simulink model "testEMplanner_cs"  (R2020b)
settings: Solver=FixedStepAuto  StartTime=0.0  StopTime=inf  FixedStep=1/1000  RelTol=1e-3
PreLoadFcn:
  | mbxruntime.callbacks.PreLoadFcn(bdroot);
PostLoadFcn:
  | mbxruntime.callbacks.PostLoadFcn(bdroot);
InitFcn:
  | mbxruntime.callbacks.InitFcn(bdroot);
StartFcn:
  | mbxruntime.callbacks.StartFcn(bdroot);
StopFcn:
  | mbxruntime.callbacks.StopFcn(bdroot);
model workspace: external: MAT-File testEMplanner_cs_hws.mat (data not in the file)
undefined symbols (not defined in the file): aubr, c_factor, cf, cr, DiscIntNeverNeededParam, global_path_x, global_path_y, KD_PID_distance, KD_PID_speed, KI_PID_distance, KI_PID_speed, KP_PID_distance, KP_PID_speed, la, lb, LQR_K1, LQR_K2, LQR_K3, LQR_K4, m, rack_displacement, right_wheel_ground, tablebr, vubr, vx_break_point
libraries: PreScanSimulinkLibrary x38, Solver_SF x1
(part 1 of 16)
CloseFcn:
  | mbxruntime.callbacks.CloseFcn(bdroot);
settings Model: Creator=PRESCAN  LastModifiedBy=iJeju
settings DataIOCC: LimitDataPoints=on  SaveFormat=Array  SignalLoggingSaveFormat=ModelDataLogs  ReturnWorkspaceOutputs=off
settings OptimizationCC: ExpressionDepthLimit=2147483647  ZeroExternalMemoryAtStartup=off  ZeroInternalMemoryAtStartup=off  InitFltsAndDblsToZero=on  LifeSpan=inf
settings DebuggingCC: SaveWithParameterizedLinksMsg=none  UnderspecifiedInitializationDetection=Classic  MergeDetectMultiDrivingBlocksExec=none  SignalResolutionControl=TryResolveAllWithWarning  MultiTaskDSMMsg=warning  MultiTaskCondExecSysMsg=none  UnderSpecifiedDataTypeMsg=warning  FcnCallInpInsideContextMsg=warning  StateNameClashWarn=warning  SFUnexpectedBacktrackingDiag=warning  SFNoUnconditionalDefaultTransitionDiag=warning  SFExecutionAtInitializationDiag=none  UnderSpecifiedDimensionMsg=warning  ArithmeticOperatorsInVariantConditions=warning
settings HardwareCC: ProdBitPerPointer=32  ProdBitPerSizeT=32  ProdBitPerPtrDiffT=32  ProdLargestAtomicFloat=None  ProdIntDivRoundTo=Undefined  ProdEndianess=Unspecified  ProdWordSize=32  ProdHWDeviceType=32-bit Generic
settings ModelReferenceCC: UpdateModelReferenceTargets=IfOutOfDate  PropagateSignalLabelsOutOfModel=off
settings SFSimCC: SimUseLocalCustomCode=off  SimParseCustomCode=off  CustomCodeUndefinedFunction=UseInterfaceOnly
settings SFSimCC: SimCustomHeaderCode=|
  | #include "prescan.h"
  | #include "prescan_platform.h"
settings RTWCC: RTWUseLocalCustomCode=off  TargetLang=C++
settings CodeAppCC: StateflowObjectComments=on
settings GRTTargetCC: TargetFcnLib=ansi_tfl_tmw.mat  TargetLangStandard=C++03 (ISO)  CodeInterfacePackaging=C++ class
settings ConfigComp: CovMetricSettings=dw  CovSaveCumulativeToWorkspaceVar=on  CovSaveSingleToWorkspaceVar=on  CovExternalEMLEnable=off

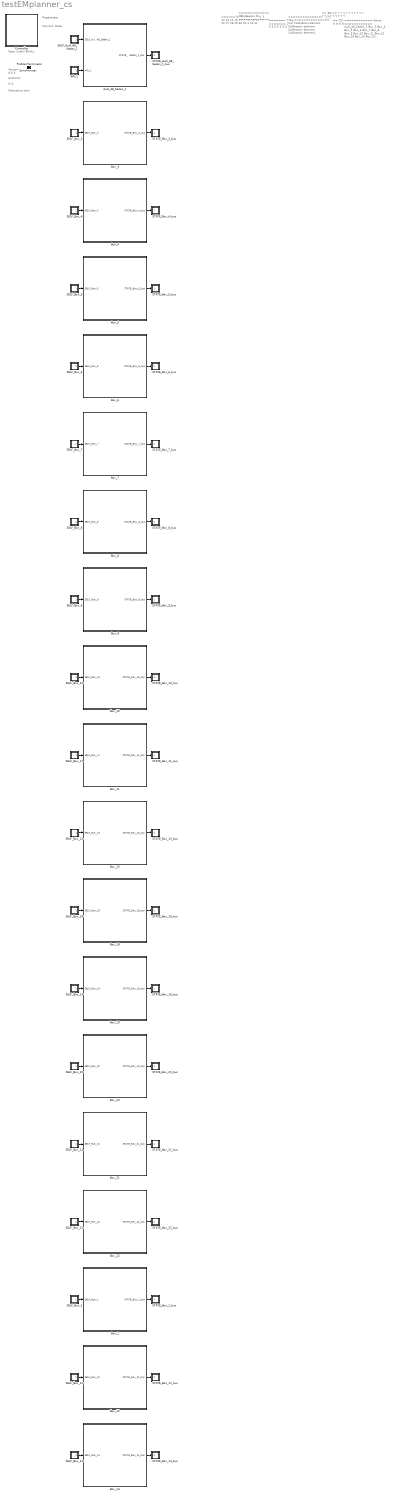
== system testEMplanner_cs ==
  note: Regenerate
  note: Simulink Mode
  note: Open Useful Blocks
  note: 8.6.0
  note: Version:
  note: Author(s):
  note: N.A.
  note: Descriptive text:
  note: ======
      | Num ID
      | ======
      | 3
      | 12
      | 13
      | 14
      | 15
      | 16
      | 17
      | 18
      | 19
      | 20
      | 22
      | 27
      | 28
      | 29
      | 30
      | 31
      | 4
      | 10
      | 21
  note: =============
      | OBU-Beacon ID
      | =============
  note: =======
      | Type ID
      | =======
      | 1
      | 5
      | 5
      | 5
      | 5
      | 5
      | 5
      | 5
      | 5
      | 5
      | 5
      | 5
      | 5
      | 5
      | 5
      | 5
      | 5
      | 5
      | 5
  note: ===============
      | Type Tag
      | ===============
      | Car
      | Calibration element
      | Calibration element
      | Calibration element
      | Calibration element
      | Calibration element
      | Calibration element
      | Calibration element
      | Calibration element
      | Calibration element
      | Calibration element
      | Calibration element
      | Calibration element
      | Calibration element
      | Calibration element
      | Calibration element
      | Calibration element
      | Calibration element
      | Calibration element
  note: ==
      | SD
      | ==
      | Y
      | Y
      | Y
      | Y
      | Y
      | Y
      | Y
      | Y
      | Y
      | Y
      | Y
      | Y
      | Y
      | Y
      | Y
      | Y
      | Y
      | Y
      | Y
  note: ==
      | CD
      | ==
      | N
      | N
      | N
      | N
      | N
      | N
      | N
      | N
      | N
      | N
      | N
      | N
      | N
      | N
      | N
      | N
      | N
      | N
      | N
  note: ============
      | Name
      | ============
      | Audi_A8_Sedan_1
      | Box_3
      | Box_4
      | Box_5
      | Box_6
      | Box_7
      | Box_8
      | Box_9
      | Box_10
      | Box_11
      | Box_13
      | Box_18
      | Box_19
      | Box_20
      | Box_21
      | Box_22
      | Box_1
      | Box_12
      | Box_14
  AIR_1 : Subsystem  Tag=sensor/AIR  Priority=3  LoadFcn=load('PrescanAIRSensorData.mat');load('PrescanAIRSensorMessage.mat')  mask(PreScan Source Block: Actor Independent Receiver (AIR)){}
      mask help:
      | The Actor Information Receiver sensor provides a fast, simple and generic detection solution which is not tied up to a specific technology. The AIR detects the intersection point of the bounding box with the straight line from the sensor axis system to the middle of the bounding box.
      |
      | For more information, please click Help.
      settings: OpenFcn=open_system([gcb '/Sensor'],'mask')
      mask Help: eval('openHelp(413)')
      mask Display: image(imread('AIR.png'))
  Audi_A8_Sedan_1 : Subsystem  Tag=WorldObjectSubSystem  InitFcn=UniqueId = '15';
      mask init:
      | modelPath = GenericModelHelper.getGenericModelFilePath('ModelDepo','Vehicles\Audi_A8\Audi_A8.pgmb','d771622804618130053427da08a6d484');imagePath = GenericModelHelper.getCompilationPicture(modelPath, 'Audi_A8_HighPoly.png');
      mask Display: image(imread(imagePath));color('white');text(0, 0, ' ID=3\n')
  Box_1 : Subsystem  Tag=WorldObjectSubSystem  InitFcn=|
      | UniqueId = '143';
      | UniqueId = '276';
      mask init:
      | imagePath=which('Box.jpg');
      mask Display: image(imread(imagePath));color('white');text(0, 0, ' ID=4\n')
  Box_10 : Subsystem  Tag=WorldObjectSubSystem  InitFcn=UniqueId = '177';
      mask init:
      | imagePath=which('Box.jpg');
      mask Display: image(imread(imagePath));color('white');text(0, 0, ' ID=19\n')
  Box_11 : Subsystem  Tag=WorldObjectSubSystem  InitFcn=UniqueId = '178';
      mask init:
      | imagePath=which('Box.jpg');
      mask Display: image(imread(imagePath));color('white');text(0, 0, ' ID=20\n')
  Box_12 : Subsystem  Tag=WorldObjectSubSystem  InitFcn=|
      | UniqueId = '179';
      | UniqueId = '277';
      mask init:
      | imagePath=which('Box.jpg');
      mask Display: image(imread(imagePath));color('white');text(0, 0, ' ID=10\n')
  Box_13 : Subsystem  Tag=WorldObjectSubSystem  InitFcn=UniqueId = '182';
      mask init:
      | imagePath=which('Box.jpg');
      mask Display: image(imread(imagePath));color('white');text(0, 0, ' ID=22\n')
  Box_14 : Subsystem  Tag=WorldObjectSubSystem  InitFcn=|
      | UniqueId = '183';
      | UniqueId = '281';
      mask init:
      | imagePath=which('Box.jpg');
      mask Display: image(imread(imagePath));color('white');text(0, 0, ' ID=21\n')
  Box_18 : Subsystem  Tag=WorldObjectSubSystem  InitFcn=UniqueId = '195';
      mask init:
      | imagePath=which('Box.jpg');
      mask Display: image(imread(imagePath));color('white');text(0, 0, ' ID=27\n')
  Box_19 : Subsystem  Tag=WorldObjectSubSystem  InitFcn=UniqueId = '196';
      mask init:
      | imagePath=which('Box.jpg');
      mask Display: image(imread(imagePath));color('white');text(0, 0, ' ID=28\n')
  Box_20 : Subsystem  Tag=WorldObjectSubSystem  InitFcn=UniqueId = '197';
      mask init:
      | imagePath=which('Box.jpg');
      mask Display: image(imread(imagePath));color('white');text(0, 0, ' ID=29\n')
  Box_21 : Subsystem  Tag=WorldObjectSubSystem  InitFcn=UniqueId = '198';
      mask init:
      | imagePath=which('Box.jpg');
      mask Display: image(imread(imagePath));color('white');text(0, 0, ' ID=30\n')
  Box_22 : Subsystem  Tag=WorldObjectSubSystem  InitFcn=UniqueId = '199';
      mask init:
      | imagePath=which('Box.jpg');
      mask Display: image(imread(imagePath));color('white');text(0, 0, ' ID=31\n')
  Box_3 : Subsystem  Tag=WorldObjectSubSystem  InitFcn=UniqueId = '170';
      mask init:
      | imagePath=which('Box.jpg');
      mask Display: image(imread(imagePath));color('white');text(0, 0, ' ID=12\n')
  Box_4 : Subsystem  Tag=WorldObjectSubSystem  InitFcn=UniqueId = '171';
      mask init:
      | imagePath=which('Box.jpg');
      mask Display: image(imread(imagePath));color('white');text(0, 0, ' ID=13\n')
  Box_5 : Subsystem  Tag=WorldObjectSubSystem  InitFcn=UniqueId = '172';
      mask init:
      | imagePath=which('Box.jpg');
      mask Display: image(imread(imagePath));color('white');text(0, 0, ' ID=14\n')
  Box_6 : Subsystem  Tag=WorldObjectSubSystem  InitFcn=UniqueId = '173';
      mask init:
      | imagePath=which('Box.jpg');
      mask Display: image(imread(imagePath));color('white');text(0, 0, ' ID=15\n')
  Box_7 : Subsystem  Tag=WorldObjectSubSystem  InitFcn=UniqueId = '174';
      mask init:
      | imagePath=which('Box.jpg');
      mask Display: image(imread(imagePath));color('white');text(0, 0, ' ID=16\n')
  Box_8 : Subsystem  Tag=WorldObjectSubSystem  InitFcn=UniqueId = '175';
      mask init:
      | imagePath=which('Box.jpg');
      mask Display: image(imread(imagePath));color('white');text(0, 0, ' ID=17\n')
  Box_9 : Subsystem  Tag=WorldObjectSubSystem  InitFcn=UniqueId = '176';
      mask init:
      | imagePath=which('Box.jpg');
      mask Display: image(imread(imagePath));color('white');text(0, 0, ' ID=18\n')
  Controller : Subsystem  Description=73E1798A8DDC6C7523B87793F8265ADBA4092B5E929CBACDAD4A169A3E9AE576  Priority=-1  LoadFcn=load PreScanControllerData  mask(PreScan Simulation Controller){prescanversion='8.6.0', ModelReferencing=off, TimeStep=50/1000, ControlMode=0, PreScanExecutionMode=on, ControllerCount=0, ControllerIndex=0, ControllerOptions=''}
      mask prompts: prescanversion "PreScan Version"; ModelReferencing "Use Model Referencing"; TimeStep "Upload Period [s]"; ControlMode "Control Mode"; PreScanExecutionMode "Execution Mode"; ControllerCount "Controller Count"; ControllerIndex "Controller Index"; ControllerOptions "Controller Options"
      mask help:
      | Please do not remove this block from the compilation sheet,
      | as it connects the model to the PreScan environment.
      mask init:
      | model = bdroot(gcb);
      | ExperimentFile = mbxruntime.findExperimentFile(model,true); %relative path
      | 
      | [d1, d2, d3, prescandata] = prescan_Settings();
      | ModelDepo = fullfile(prescandata,'ModelDepo'); 
      | 
      | RTmode = mbxruntime.getRTMode(model);
      | 
      | SimulationMode = get_param(bdroot,'SimulationMode');
      | if strcmp(SimulationMode, 'rapid-accelerator')
      |     SimulationMode = 'external';
      | end
      | TargetName = get_param(bdroot,'SystemTargetFile');
      settings: ModelCloseFcn=assignin('base',['model_closed_' bdroot],true);
      mask Help: eval('openHelp(812)')
      mask Display: image(imread('prescanlogo.ico'))
  PreScanTerminator : Subsystem  Tag=PreScanTerminator  Priority=999  LoadFcn=load PrescanTerminatorData  mask(PreScan Simulation Terminator){TimeStep=50/1000}
      mask prompts: TimeStep "Upload Period [s]"
      mask help:
      | Please do not remove this block from the compilation sheet as it
      | connects the model to the PreScan environment.
      mask Help: eval('openHelp(812)')
      mask Display: image(imread('prescanlogo.ico'))
  SELF_Audi_A8_Sedan_1 : Subsystem  Tag=sensor/SelfPort  Priority=3  LoadFcn=load('PreScanSelfSensorData.mat')  mask(PreScan Source Block: SELF){}
      mask help:
      | The SELF port shows (state) information of the actor itself. The outputs are position in the experiment's axis system and the GPS coordinates, and the object's absolute velocity and compass heading.
      |
      | For more information, please click Help.
      settings: OpenFcn=open_system([gcb '/Sensor'],'mask')
      mask Help: eval('openHelp(462)')
      mask Display: image(imread('GPS.png'))
  SELF_Box_1 : Subsystem  Tag=sensor/SelfPort  Priority=3  LoadFcn=load('PreScanSelfSensorData.mat')  mask(PreScan Source Block: SELF){}
      mask help:
      | The SELF port shows (state) information of the actor itself. The outputs are position in the experiment's axis system and the GPS coordinates, and the object's absolute velocity and compass heading.
      |
      | For more information, please click Help.
      settings: OpenFcn=open_system([gcb '/Sensor'],'mask')
      mask Help: eval('openHelp(462)')
      mask Display: image(imread('GPS.png'))
  SELF_Box_10 : Subsystem  Tag=sensor/SelfPort  Priority=3  LoadFcn=load('PreScanSelfSensorData.mat')  mask(PreScan Source Block: SELF){}
      mask help:
      | The SELF port shows (state) information of the actor itself. The outputs are position in the experiment's axis system and the GPS coordinates, and the object's absolute velocity and compass heading.
      |
      | For more information, please click Help.
      settings: OpenFcn=open_system([gcb '/Sensor'],'mask')
      mask Help: eval('openHelp(462)')
      mask Display: image(imread('GPS.png'))
  SELF_Box_11 : Subsystem  Tag=sensor/SelfPort  Priority=3  LoadFcn=load('PreScanSelfSensorData.mat')  mask(PreScan Source Block: SELF){}
      mask help:
      | The SELF port shows (state) information of the actor itself. The outputs are position in the experiment's axis system and the GPS coordinates, and the object's absolute velocity and compass heading.
      |
      | For more information, please click Help.
      settings: OpenFcn=open_system([gcb '/Sensor'],'mask')
      mask Help: eval('openHelp(462)')
      mask Display: image(imread('GPS.png'))
  SELF_Box_12 : Subsystem  Tag=sensor/SelfPort  Priority=3  LoadFcn=load('PreScanSelfSensorData.mat')  mask(PreScan Source Block: SELF){}
      mask help:
      | The SELF port shows (state) information of the actor itself. The outputs are position in the experiment's axis system and the GPS coordinates, and the object's absolute velocity and compass heading.
      |
      | For more information, please click Help.
      settings: OpenFcn=open_system([gcb '/Sensor'],'mask')
      mask Help: eval('openHelp(462)')
      mask Display: image(imread('GPS.png'))
  SELF_Box_13 : Subsystem  Tag=sensor/SelfPort  Priority=3  LoadFcn=load('PreScanSelfSensorData.mat')  mask(PreScan Source Block: SELF){}
      mask help:
      | The SELF port shows (state) information of the actor itself. The outputs are position in the experiment's axis system and the GPS coordinates, and the object's absolute velocity and compass heading.
      |
      | For more information, please click Help.
      settings: OpenFcn=open_system([gcb '/Sensor'],'mask')
      mask Help: eval('openHelp(462)')
      mask Display: image(imread('GPS.png'))
  SELF_Box_14 : Subsystem  Tag=sensor/SelfPort  Priority=3  LoadFcn=load('PreScanSelfSensorData.mat')  mask(PreScan Source Block: SELF){}
      mask help:
      | The SELF port shows (state) information of the actor itself. The outputs are position in the experiment's axis system and the GPS coordinates, and the object's absolute velocity and compass heading.
      |
      | For more information, please click Help.
      settings: OpenFcn=open_system([gcb '/Sensor'],'mask')
      mask Help: eval('openHelp(462)')
      mask Display: image(imread('GPS.png'))
  SELF_Box_18 : Subsystem  Tag=sensor/SelfPort  Priority=3  LoadFcn=load('PreScanSelfSensorData.mat')  mask(PreScan Source Block: SELF){}
      mask help:
      | The SELF port shows (state) information of the actor itself. The outputs are position in the experiment's axis system and the GPS coordinates, and the object's absolute velocity and compass heading.
      |
      | For more information, please click Help.
      settings: OpenFcn=open_system([gcb '/Sensor'],'mask')
      mask Help: eval('openHelp(462)')
      mask Display: image(imread('GPS.png'))
  SELF_Box_19 : Subsystem  Tag=sensor/SelfPort  Priority=3  LoadFcn=load('PreScanSelfSensorData.mat')  mask(PreScan Source Block: SELF){}
      mask help:
      | The SELF port shows (state) information of the actor itself. The outputs are position in the experiment's axis system and the GPS coordinates, and the object's absolute velocity and compass heading.
      |
      | For more information, please click Help.
      settings: OpenFcn=open_system([gcb '/Sensor'],'mask')
      mask Help: eval('openHelp(462)')
      mask Display: image(imread('GPS.png'))
  SELF_Box_20 : Subsystem  Tag=sensor/SelfPort  Priority=3  LoadFcn=load('PreScanSelfSensorData.mat')  mask(PreScan Source Block: SELF){}
      mask help:
      | The SELF port shows (state) information of the actor itself. The outputs are position in the experiment's axis system and the GPS coordinates, and the object's absolute velocity and compass heading.
      |
      | For more information, please click Help.
      settings: OpenFcn=open_system([gcb '/Sensor'],'mask')
      mask Help: eval('openHelp(462)')
      mask Display: image(imread('GPS.png'))
  SELF_Box_21 : Subsystem  Tag=sensor/SelfPort  Priority=3  LoadFcn=load('PreScanSelfSensorData.mat')  mask(PreScan Source Block: SELF){}
      mask help:
      | The SELF port shows (state) information of the actor itself. The outputs are position in the experiment's axis system and the GPS coordinates, and the object's absolute velocity and compass heading.
      |
      | For more information, please click Help.
      settings: OpenFcn=open_system([gcb '/Sensor'],'mask')
      mask Help: eval('openHelp(462)')
      mask Display: image(imread('GPS.png'))
  SELF_Box_22 : Subsystem  Tag=sensor/SelfPort  Priority=3  LoadFcn=load('PreScanSelfSensorData.mat')  mask(PreScan Source Block: SELF){}
      mask help:
      | The SELF port shows (state) information of the actor itself. The outputs are position in the experiment's axis system and the GPS coordinates, and the object's absolute velocity and compass heading.
      |
      | For more information, please click Help.
      settings: OpenFcn=open_system([gcb '/Sensor'],'mask')
      mask Help: eval('openHelp(462)')
      mask Display: image(imread('GPS.png'))
  SELF_Box_3 : Subsystem  Tag=sensor/SelfPort  Priority=3  LoadFcn=load('PreScanSelfSensorData.mat')  mask(PreScan Source Block: SELF){}
      mask help:
      | The SELF port shows (state) information of the actor itself. The outputs are position in the experiment's axis system and the GPS coordinates, and the object's absolute velocity and compass heading.
      |
      | For more information, please click Help.
      settings: OpenFcn=open_system([gcb '/Sensor'],'mask')
      mask Help: eval('openHelp(462)')
      mask Display: image(imread('GPS.png'))
  SELF_Box_4 : Subsystem  Tag=sensor/SelfPort  Priority=3  LoadFcn=load('PreScanSelfSensorData.mat')  mask(PreScan Source Block: SELF){}
      mask help:
      | The SELF port shows (state) information of the actor itself. The outputs are position in the experiment's axis system and the GPS coordinates, and the object's absolute velocity and compass heading.
      |
      | For more information, please click Help.
      settings: OpenFcn=open_system([gcb '/Sensor'],'mask')
      mask Help: eval('openHelp(462)')
      mask Display: image(imread('GPS.png'))
  SELF_Box_5 : Subsystem  Tag=sensor/SelfPort  Priority=3  LoadFcn=load('PreScanSelfSensorData.mat')  mask(PreScan Source Block: SELF){}
      mask help:
      | The SELF port shows (state) information of the actor itself. The outputs are position in the experiment's axis system and the GPS coordinates, and the object's absolute velocity and compass heading.
      |
      | For more information, please click Help.
      settings: OpenFcn=open_system([gcb '/Sensor'],'mask')
      mask Help: eval('openHelp(462)')
      mask Display: image(imread('GPS.png'))
  SELF_Box_6 : Subsystem  Tag=sensor/SelfPort  Priority=3  LoadFcn=load('PreScanSelfSensorData.mat')  mask(PreScan Source Block: SELF){}
      mask help:
      | The SELF port shows (state) information of the actor itself. The outputs are position in the experiment's axis system and the GPS coordinates, and the object's absolute velocity and compass heading.
      |
      | For more information, please click Help.
      settings: OpenFcn=open_system([gcb '/Sensor'],'mask')
      mask Help: eval('openHelp(462)')
      mask Display: image(imread('GPS.png'))
  SELF_Box_7 : Subsystem  Tag=sensor/SelfPort  Priority=3  LoadFcn=load('PreScanSelfSensorData.mat')  mask(PreScan Source Block: SELF){}
      mask help:
      | The SELF port shows (state) information of the actor itself. The outputs are position in the experiment's axis system and the GPS coordinates, and the object's absolute velocity and compass heading.
      |
      | For more information, please click Help.
      settings: OpenFcn=open_system([gcb '/Sensor'],'mask')
      mask Help: eval('openHelp(462)')
      mask Display: image(imread('GPS.png'))
  SELF_Box_8 : Subsystem  Tag=sensor/SelfPort  Priority=3  LoadFcn=load('PreScanSelfSensorData.mat')  mask(PreScan Source Block: SELF){}
      mask help:
      | The SELF port shows (state) information of the actor itself. The outputs are position in the experiment's axis system and the GPS coordinates, and the object's absolute velocity and compass heading.
      |
      | For more information, please click Help.
      settings: OpenFcn=open_system([gcb '/Sensor'],'mask')
      mask Help: eval('openHelp(462)')
      mask Display: image(imread('GPS.png'))
  SELF_Box_9 : Subsystem  Tag=sensor/SelfPort  Priority=3  LoadFcn=load('PreScanSelfSensorData.mat')  mask(PreScan Source Block: SELF){}
      mask help:
      | The SELF port shows (state) information of the actor itself. The outputs are position in the experiment's axis system and the GPS coordinates, and the object's absolute velocity and compass heading.
      |
      | For more information, please click Help.
      settings: OpenFcn=open_system([gcb '/Sensor'],'mask')
      mask Help: eval('openHelp(462)')
      mask Display: image(imread('GPS.png'))
  STATE_Audi_A8_Sedan_1_bus : Subsystem  Tag=actuator/StatePort  Priority=0  LoadFcn=load('PreScanStateActuatorData.mat')  mask(PreScan Sink Block: State){}
      mask help:
      | The Actor State contains a vector signal of size (9x1), containing the following signals:
      |
      | -  Position    	(x,y,z)             	[m]
      | -  Velocity    	(vx,vy,vz)         	[m/s]
      | -  Angles       	(Roll, Pitch, Yaw)	[rad]
      |
      | The Actor state is defined in the global axis system.
      | The state is superponed on the Initial position defined in the GUI.
      |
      | For more information, please click Help.
      settings: OpenFcn=open_system([gcb '/Actuator'],'mask')
      mask Help: eval('openHelp(222)')
      mask Display: image(imread('State.png'))
  STATE_Box_10_bus : Subsystem  Tag=actuator/StatePort  Priority=0  LoadFcn=load('PreScanStateActuatorData.mat')  mask(PreScan Sink Block: State){}
      mask help:
      | The Actor State contains a vector signal of size (9x1), containing the following signals:
      |
      | -  Position    	(x,y,z)             	[m]
      | -  Velocity    	(vx,vy,vz)         	[m/s]
      | -  Angles       	(Roll, Pitch, Yaw)	[rad]
      |
      | The Actor state is defined in the global axis system.
      | The state is superponed on the Initial position defined in the GUI.
      |
      | For more information, please click Help.
      settings: OpenFcn=open_system([gcb '/Actuator'],'mask')
      mask Help: eval('openHelp(222)')
      mask Display: image(imread('State.png'))
  STATE_Box_11_bus : Subsystem  Tag=actuator/StatePort  Priority=0  LoadFcn=load('PreScanStateActuatorData.mat')  mask(PreScan Sink Block: State){}
      mask help:
      | The Actor State contains a vector signal of size (9x1), containing the following signals:
      |
      | -  Position    	(x,y,z)             	[m]
      | -  Velocity    	(vx,vy,vz)         	[m/s]
      | -  Angles       	(Roll, Pitch, Yaw)	[rad]
      |
      | The Actor state is defined in the global axis system.
      | The state is superponed on the Initial position defined in the GUI.
      |
      | For more information, please click Help.
      settings: OpenFcn=open_system([gcb '/Actuator'],'mask')
      mask Help: eval('openHelp(222)')
      mask Display: image(imread('State.png'))
  STATE_Box_12_bus : Subsystem  Tag=actuator/StatePort  Priority=0  LoadFcn=load('PreScanStateActuatorData.mat')  mask(PreScan Sink Block: State){}
      mask help:
      | The Actor State contains a vector signal of size (9x1), containing the following signals:
      |
      | -  Position    	(x,y,z)             	[m]
      | -  Velocity    	(vx,vy,vz)         	[m/s]
      | -  Angles       	(Roll, Pitch, Yaw)	[rad]
      |
      | The Actor state is defined in the global axis system.
      | The state is superponed on the Initial position defined in the GUI.
      |
      | For more information, please click Help.
      settings: OpenFcn=open_system([gcb '/Actuator'],'mask')
      mask Help: eval('openHelp(222)')
      mask Display: image(imread('State.png'))
  STATE_Box_13_bus : Subsystem  Tag=actuator/StatePort  Priority=0  LoadFcn=load('PreScanStateActuatorData.mat')  mask(PreScan Sink Block: State){}
      mask help:
      | The Actor State contains a vector signal of size (9x1), containing the following signals:
      |
      | -  Position    	(x,y,z)             	[m]
      | -  Velocity    	(vx,vy,vz)         	[m/s]
      | -  Angles       	(Roll, Pitch, Yaw)	[rad]
      |
      | The Actor state is defined in the global axis system.
      | The state is superponed on the Initial position defined in the GUI.
      |
      | For more information, please click Help.
      settings: OpenFcn=open_system([gcb '/Actuator'],'mask')
      mask Help: eval('openHelp(222)')
      mask Display: image(imread('State.png'))
  STATE_Box_14_bus : Subsystem  Tag=actuator/StatePort  Priority=0  LoadFcn=load('PreScanStateActuatorData.mat')  mask(PreScan Sink Block: State){}
      mask help:
      | The Actor State contains a vector signal of size (9x1), containing the following signals:
      |
      | -  Position    	(x,y,z)             	[m]
      | -  Velocity    	(vx,vy,vz)         	[m/s]
      | -  Angles       	(Roll, Pitch, Yaw)	[rad]
      |
      | The Actor state is defined in the global axis system.
      | The state is superponed on the Initial position defined in the GUI.
      |
      | For more information, please click Help.
      settings: OpenFcn=open_system([gcb '/Actuator'],'mask')
      mask Help: eval('openHelp(222)')
      mask Display: image(imread('State.png'))
  STATE_Box_18_bus : Subsystem  Tag=actuator/StatePort  Priority=0  LoadFcn=load('PreScanStateActuatorData.mat')  mask(PreScan Sink Block: State){}
      mask help:
      | The Actor State contains a vector signal of size (9x1), containing the following signals:
      |
      | -  Position    	(x,y,z)             	[m]
      | -  Velocity    	(vx,vy,vz)         	[m/s]
      | -  Angles       	(Roll, Pitch, Yaw)	[rad]
      |
      | The Actor state is defined in the global axis system.
      | The state is superponed on the Initial position defined in the GUI.
      |
      | For more information, please click Help.
      settings: OpenFcn=open_system([gcb '/Actuator'],'mask')
      mask Help: eval('openHelp(222)')
      mask Display: image(imread('State.png'))
  STATE_Box_19_bus : Subsystem  Tag=actuator/StatePort  Priority=0  LoadFcn=load('PreScanStateActuatorData.mat')  mask(PreScan Sink Block: State){}
      mask help:
      | The Actor State contains a vector signal of size (9x1), containing the following signals:
      |
      | -  Position    	(x,y,z)             	[m]
      | -  Velocity    	(vx,vy,vz)         	[m/s]
      | -  Angles       	(Roll, Pitch, Yaw)	[rad]
      |
      | The Actor state is defined in the global axis system.
      | The state is superponed on the Initial position defined in the GUI.
      |
      | For more information, please click Help.
      settings: OpenFcn=open_system([gcb '/Actuator'],'mask')
      mask Help: eval('openHelp(222)')
      mask Display: image(imread('State.png'))
  STATE_Box_1_bus : Subsystem  Tag=actuator/StatePort  Priority=0  LoadFcn=load('PreScanStateActuatorData.mat')  mask(PreScan Sink Block: State){}
      mask help:
      | The Actor State contains a vector signal of size (9x1), containing the following signals:
      |
      | -  Position    	(x,y,z)             	[m]
      | -  Velocity    	(vx,vy,vz)         	[m/s]
      | -  Angles       	(Roll, Pitch, Yaw)	[rad]
      |
      | The Actor state is defined in the global axis system.
      | The state is superponed on the Initial position defined in the GUI.
      |
      | For more information, please click Help.
      settings: OpenFcn=open_system([gcb '/Actuator'],'mask')
      mask Help: eval('openHelp(222)')
      mask Display: image(imread('State.png'))
  STATE_Box_20_bus : Subsystem  Tag=actuator/StatePort  Priority=0  LoadFcn=load('PreScanStateActuatorData.mat')  mask(PreScan Sink Block: State){}
      mask help:
      | The Actor State contains a vector signal of size (9x1), containing the following signals:
      |
      | -  Position    	(x,y,z)             	[m]
      | -  Velocity    	(vx,vy,vz)         	[m/s]
      | -  Angles       	(Roll, Pitch, Yaw)	[rad]
      |
      | The Actor state is defined in the global axis system.
      | The state is superponed on the Initial position defined in the GUI.
      |
      | For more information, please click Help.
      settings: OpenFcn=open_system([gcb '/Actuator'],'mask')
      mask Help: eval('openHelp(222)')
      mask Display: image(imread('State.png'))
  STATE_Box_21_bus : Subsystem  Tag=actuator/StatePort  Priority=0  LoadFcn=load('PreScanStateActuatorData.mat')  mask(PreScan Sink Block: State){}
      mask help:
      | The Actor State contains a vector signal of size (9x1), containing the following signals:
      |
      | -  Position    	(x,y,z)             	[m]
      | -  Velocity    	(vx,vy,vz)         	[m/s]
      | -  Angles       	(Roll, Pitch, Yaw)	[rad]
      |
      | The Actor state is defined in the global axis system.
      | The state is superponed on the Initial position defined in the GUI.
      |
      | For more information, please click Help.
      settings: OpenFcn=open_system([gcb '/Actuator'],'mask')
      mask Help: eval('openHelp(222)')
      mask Display: image(imread('State.png'))
  STATE_Box_22_bus : Subsystem  Tag=actuator/StatePort  Priority=0  LoadFcn=load('PreScanStateActuatorData.mat')  mask(PreScan Sink Block: State){}
      mask help:
      | The Actor State contains a vector signal of size (9x1), containing the following signals:
      |
      | -  Position    	(x,y,z)             	[m]
      | -  Velocity    	(vx,vy,vz)         	[m/s]
      | -  Angles       	(Roll, Pitch, Yaw)	[rad]
      |
      | The Actor state is defined in the global axis system.
      | The state is superponed on the Initial position defined in the GUI.
      |
      | For more information, please click Help.
      settings: OpenFcn=open_system([gcb '/Actuator'],'mask')
      mask Help: eval('openHelp(222)')
      mask Display: image(imread('State.png'))
  STATE_Box_3_bus : Subsystem  Tag=actuator/StatePort  Priority=0  LoadFcn=load('PreScanStateActuatorData.mat')  mask(PreScan Sink Block: State){}
      mask help:
      | The Actor State contains a vector signal of size (9x1), containing the following signals:
      |
      | -  Position    	(x,y,z)             	[m]
      | -  Velocity    	(vx,vy,vz)         	[m/s]
      | -  Angles       	(Roll, Pitch, Yaw)	[rad]
      |
      | The Actor state is defined in the global axis system.
      | The state is superponed on the Initial position defined in the GUI.
      |
      | For more information, please click Help.
      settings: OpenFcn=open_system([gcb '/Actuator'],'mask')
      mask Help: eval('openHelp(222)')
      mask Display: image(imread('State.png'))
  STATE_Box_4_bus : Subsystem  Tag=actuator/StatePort  Priority=0  LoadFcn=load('PreScanStateActuatorData.mat')  mask(PreScan Sink Block: State){}
      mask help:
      | The Actor State contains a vector signal of size (9x1), containing the following signals:
      |
      | -  Position    	(x,y,z)             	[m]
      | -  Velocity    	(vx,vy,vz)         	[m/s]
      | -  Angles       	(Roll, Pitch, Yaw)	[rad]
      |
      | The Actor state is defined in the global axis system.
      | The state is superponed on the Initial position defined in the GUI.
      |
      | For more information, please click Help.
      settings: OpenFcn=open_system([gcb '/Actuator'],'mask')
      mask Help: eval('openHelp(222)')
      mask Display: image(imread('State.png'))
  STATE_Box_5_bus : Subsystem  Tag=actuator/StatePort  Priority=0  LoadFcn=load('PreScanStateActuatorData.mat')  mask(PreScan Sink Block: State){}
      mask help:
      | The Actor State contains a vector signal of size (9x1), containing the following signals:
      |
      | -  Position    	(x,y,z)             	[m]
      | -  Velocity    	(vx,vy,vz)         	[m/s]
      | -  Angles       	(Roll, Pitch, Yaw)	[rad]
      |
      | The Actor state is defined in the global axis system.
      | The state is superponed on the Initial position defined in the GUI.
      |
      | For more information, please click Help.
      settings: OpenFcn=open_system([gcb '/Actuator'],'mask')
      mask Help: eval('openHelp(222)')
      mask Display: image(imread('State.png'))
  STATE_Box_6_bus : Subsystem  Tag=actuator/StatePort  Priority=0  LoadFcn=load('PreScanStateActuatorData.mat')  mask(PreScan Sink Block: State){}
      mask help:
      | The Actor State contains a vector signal of size (9x1), containing the following signals:
      |
      | -  Position    	(x,y,z)             	[m]
      | -  Velocity    	(vx,vy,vz)         	[m/s]
      | -  Angles       	(Roll, Pitch, Yaw)	[rad]
      |
      | The Actor state is defined in the global axis system.
      | The state is superponed on the Initial position defined in the GUI.
      |
      | For more information, please click Help.
      settings: OpenFcn=open_system([gcb '/Actuator'],'mask')
      mask Help: eval('openHelp(222)')
      mask Display: image(imread('State.png'))
  STATE_Box_7_bus : Subsystem  Tag=actuator/StatePort  Priority=0  LoadFcn=load('PreScanStateActuatorData.mat')  mask(PreScan Sink Block: State){}
      mask help:
      | The Actor State contains a vector signal of size (9x1), containing the following signals:
      |
      | -  Position    	(x,y,z)             	[m]
      | -  Velocity    	(vx,vy,vz)         	[m/s]
      | -  Angles       	(Roll, Pitch, Yaw)	[rad]
      |
      | The Actor state is defined in the global axis system.
      | The state is superponed on the Initial position defined in the GUI.
      |
      | For more information, please click Help.
      settings: OpenFcn=open_system([gcb '/Actuator'],'mask')
      mask Help: eval('openHelp(222)')
      mask Display: image(imread('State.png'))
  STATE_Box_8_bus : Subsystem  Tag=actuator/StatePort  Priority=0  LoadFcn=load('PreScanStateActuatorData.mat')  mask(PreScan Sink Block: State){}
      mask help:
      | The Actor State contains a vector signal of size (9x1), containing the following signals:
      |
      | -  Position    	(x,y,z)             	[m]
      | -  Velocity    	(vx,vy,vz)         	[m/s]
      | -  Angles       	(Roll, Pitch, Yaw)	[rad]
      |
      | The Actor state is defined in the global axis system.
      | The state is superponed on the Initial position defined in the GUI.
      |
      | For more information, please click Help.
      settings: OpenFcn=open_system([gcb '/Actuator'],'mask')
      mask Help: eval('openHelp(222)')
      mask Display: image(imread('State.png'))
  STATE_Box_9_bus : Subsystem  Tag=actuator/StatePort  Priority=0  LoadFcn=load('PreScanStateActuatorData.mat')  mask(PreScan Sink Block: State){}
      mask help:
      | The Actor State contains a vector signal of size (9x1), containing the following signals:
      |
      | -  Position    	(x,y,z)             	[m]
      | -  Velocity    	(vx,vy,vz)         	[m/s]
      | -  Angles       	(Roll, Pitch, Yaw)	[rad]
      |
      | The Actor state is defined in the global axis system.
      | The state is superponed on the Initial position defined in the GUI.
      |
      | For more information, please click Help.
      settings: OpenFcn=open_system([gcb '/Actuator'],'mask')
      mask Help: eval('openHelp(222)')
      mask Display: image(imread('State.png'))
  Synchronizer : Subsystem  Tag=PreScanSynchronizer  Priority=1  LoadFcn=load PrescanSynchronizeData  mask(PreScan Simulation Core Block){TimeStep=50/1000}
      mask prompts: TimeStep "Timestep [s]"
      mask help:
      | Please do not remove this block from the PreScan compilation sheet,
      | as it contains essential configuration parameters for a PreScan simulation.
      settings: DeleteFcn=PreScanBlockDeleteFcn;
      mask Display: image(imread('prescanlogo.ico'))
  wires:
  Audi_A8_Sedan_1/1(STATE_Audi_A8_Sedan_1_bus) -> STATE_Audi_A8_Sedan_1_bus/1(STATE_Audi_A8_Sedan_1_bus)
  SELF_Audi_A8_Sedan_1/1(SELF_Audi_A8_Sedan_1) -> Audi_A8_Sedan_1/1(SELF_Audi_A8_Sedan_1)
  AIR_1/1(AIR_1) -> Audi_A8_Sedan_1/2(AIR_1)
  Box_1/1(STATE_Box_1_bus) -> STATE_Box_1_bus/1(STATE_Box_1_bus)
  SELF_Box_1/1(SELF_Box_1) -> Box_1/1(SELF_Box_1)
  Box_3/1(STATE_Box_3_bus) -> STATE_Box_3_bus/1(STATE_Box_3_bus)
  SELF_Box_3/1(SELF_Box_3) -> Box_3/1(SELF_Box_3)
  Box_4/1(STATE_Box_4_bus) -> STATE_Box_4_bus/1(STATE_Box_4_bus)
  SELF_Box_4/1(SELF_Box_4) -> Box_4/1(SELF_Box_4)
  Box_5/1(STATE_Box_5_bus) -> STATE_Box_5_bus/1(STATE_Box_5_bus)
  SELF_Box_5/1(SELF_Box_5) -> Box_5/1(SELF_Box_5)
  Box_6/1(STATE_Box_6_bus) -> STATE_Box_6_bus/1(STATE_Box_6_bus)
  SELF_Box_6/1(SELF_Box_6) -> Box_6/1(SELF_Box_6)
  Box_7/1(STATE_Box_7_bus) -> STATE_Box_7_bus/1(STATE_Box_7_bus)
  SELF_Box_7/1(SELF_Box_7) -> Box_7/1(SELF_Box_7)
  Box_8/1(STATE_Box_8_bus) -> STATE_Box_8_bus/1(STATE_Box_8_bus)
  SELF_Box_8/1(SELF_Box_8) -> Box_8/1(SELF_Box_8)
  Box_9/1(STATE_Box_9_bus) -> STATE_Box_9_bus/1(STATE_Box_9_bus)
  SELF_Box_9/1(SELF_Box_9) -> Box_9/1(SELF_Box_9)
  Box_10/1(STATE_Box_10_bus) -> STATE_Box_10_bus/1(STATE_Box_10_bus)
  SELF_Box_10/1(SELF_Box_10) -> Box_10/1(SELF_Box_10)
  Box_11/1(STATE_Box_11_bus) -> STATE_Box_11_bus/1(STATE_Box_11_bus)
  SELF_Box_11/1(SELF_Box_11) -> Box_11/1(SELF_Box_11)
  Box_12/1(STATE_Box_12_bus) -> STATE_Box_12_bus/1(STATE_Box_12_bus)
  SELF_Box_12/1(SELF_Box_12) -> Box_12/1(SELF_Box_12)
  Box_13/1(STATE_Box_13_bus) -> STATE_Box_13_bus/1(STATE_Box_13_bus)
  SELF_Box_13/1(SELF_Box_13) -> Box_13/1(SELF_Box_13)
  Box_14/1(STATE_Box_14_bus) -> STATE_Box_14_bus/1(STATE_Box_14_bus)
  SELF_Box_14/1(SELF_Box_14) -> Box_14/1(SELF_Box_14)
  Box_18/1(STATE_Box_18_bus) -> STATE_Box_18_bus/1(STATE_Box_18_bus)
  SELF_Box_18/1(SELF_Box_18) -> Box_18/1(SELF_Box_18)
  Box_19/1(STATE_Box_19_bus) -> STATE_Box_19_bus/1(STATE_Box_19_bus)
  SELF_Box_19/1(SELF_Box_19) -> Box_19/1(SELF_Box_19)
  Box_20/1(STATE_Box_20_bus) -> STATE_Box_20_bus/1(STATE_Box_20_bus)
  SELF_Box_20/1(SELF_Box_20) -> Box_20/1(SELF_Box_20)
  Box_21/1(STATE_Box_21_bus) -> STATE_Box_21_bus/1(STATE_Box_21_bus)
  SELF_Box_21/1(SELF_Box_21) -> Box_21/1(SELF_Box_21)
  Box_22/1(STATE_Box_22_bus) -> STATE_Box_22_bus/1(STATE_Box_22_bus)
  SELF_Box_22/1(SELF_Box_22) -> Box_22/1(SELF_Box_22)

== system testEMplanner_cs/AIR_1 ==
  Sensor : S-Function  FunctionName=sfun_AIRSensor  Parameters=detectableObjects, sensorID, timestep  SFunctionDeploymentMode=off  EnableBusSupport=off  mask(PreScan Source Block: Actor Independent Receiver (AIR)){detectableObjects=32, sensorID=142, timestep=50/1000}
      mask prompts: detectableObjects "Max detectable objects"; sensorID "Sensor ID"; timestep "MATLAB timestep:"
      mask help:
      | The Actor Information Receiver sensor provides a fast, simple and generic detection solution which is not tied up to a specific technology. The AIR detects the intersection point of the bounding box with the straight line from the sensor axis system to the middle of the bounding box.
      |
      | For more information, please click Help.
      mask Help: eval('openHelp(413)')
      mask Display: image(imread('AIR.png'))
  AIR_1 : Outport  Tag=outport/AIR  OutDataTypeStr=Bus: PRESCAN_AIRSENSORMESSAGE  PortDimensions=32  SampleTime=50/1000
  wires:
  Sensor/1 -> AIR_1/1

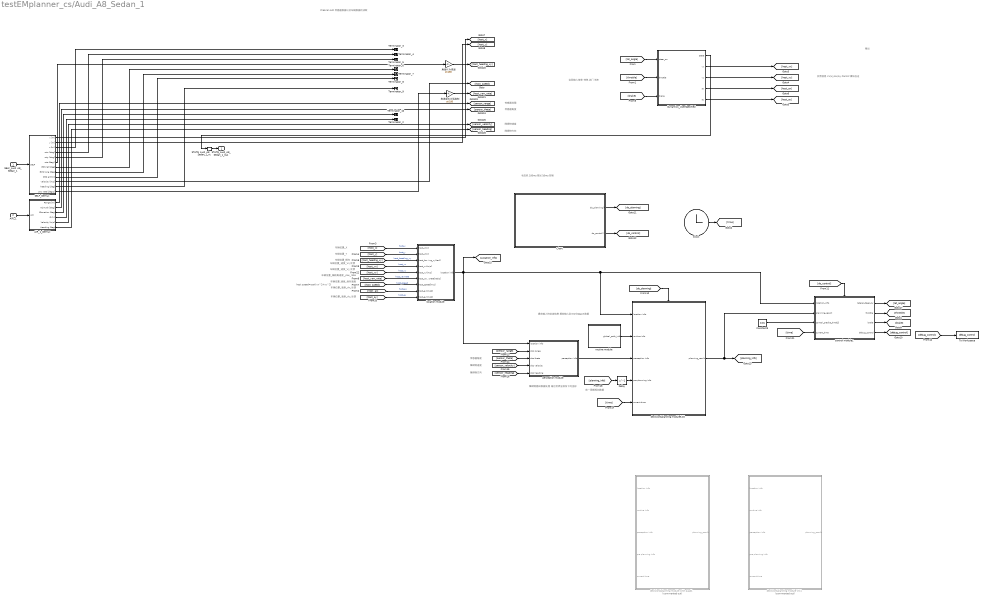
== system testEMplanner_cs/Audi_A8_Sedan_1 ==
  note: 传感器范围
  note: 输出
  note: host speed=sqrt(vx^2+vy^2)
  note: 反馈信息
      | Vx/Vy/Ax/Ay
      | Carsim模块在这
  note: Prescan AIR
      | 传感器数据以及车辆数据的读取
  note: 状态机
      | 100ms规划/10ms控制
  note: 传感器角度
  note: 障碍物速度
  note: 障碍物方向
  note: 实际输入信息
      | 转角/油门/刹车
  note: 车辆位置_X
  note: 车辆位置_Y
  note: 车辆位置_朝向
  note: 车辆位置_速度_Vx_反馈
  note: 车辆位置_速度_Vy_反馈
  note: 车辆位置_偏航角速度_yaw_rate
  note: 车辆位置_速度_绝对速度
  note: 车辆位置_速度_Ay_反馈
  note: 车辆位置_速度_Ax_反馈
  note: 前一周期规划数据
  note: 障碍物速度
  note: 传感器角度
  note: 障碍物方向
  note: 障碍物感知数据处理
      | 输出世界坐标系下的坐标
  note: 提前输入的轨迹信息
      | 提前输入到WorkSpace数据
  SELF_Audi_A8_Sedan_1 : Inport  Tag=inport/SelfPort  OutDataTypeStr=Bus: PRESCAN_SELFSENSORDATA  PortDimensions=1  SampleTime=50/1000  BusOutputAsStruct=on
  AIR_1 : Inport  Tag=inport/AIR  Port=2  OutDataTypeStr=Bus: PRESCAN_AIRSENSORMESSAGE  PortDimensions=32  SampleTime=50/1000  BusOutputAsStruct=on
  AIR_1_Demux : Subsystem  Tag=demux/AIR  mask(PreScan Demux Block: AIR){DetectionType=Center, detectableObjects=32}
      mask prompts: DetectionType "Detection Type"; detectableObjects "Max. detectable objects"
      mask help:
      | The Actor Information Receiver sensor provides a fast, simple and generic detection solution which is not tied up to a specific technology and can be used for scenarios in which a simple sensor is needed.
      |
      | For more information, please click Help.
      mask init:
      | switch DetectionType
      |     case 1
      |         DetectionTypeStr = 'Center';
      |     case 2
      |         DetectionTypeStr = 'BBox';
      |     case 3
      |         DetectionTypeStr = 'CoG';
      |     otherwise
      |         DetectionTypeStr = 'Unknown';
      | end
      settings: DeleteFcn=PreScanBlockDeleteFcn;
      mask Help: eval('openHelp(413)')
      mask TypeOptions DetectionType: Center | BBox | CoG
      mask Display:
      | disp(char('Det. type:         ',['{\it',DetectionTypeStr,'}']),'texmode','on')
      | port_label('output',1,'Range [m]')
      | port_label('output',2,'{\theta} [deg]','texmode','on')
      | port_label('output',3,'{\phi} [deg]','texmode','on')
      | port_label('output',4,'ID [-]','texmode','on')
      | port_label('output',5,'Velocity [m/s]','texmode','on')
      | port_label('output',6,'Heading [deg]','texmode','on')
  Chart : Stateflow chart  TreatAsAtomicUnit=on
  Clock : Clock
  Constant3 : Constant  Value=0.01
  Delay : Delay  DelayLength=1
  Dynamics_UserSpecified : Subsystem  Tag=UserSpecified_Subsys  Description=.\Caisim-1\Extensions\Simulink\CarSim_VehicleDynamics.mdl  mask(User specified subsystem){update=off, sourcefilename=.\Caisim-1\Extensions\Simulink\CarSim_VehicleDynamics.mdl}
      mask prompts: update "Update (default: not checked)"; sourcefilename "Source file name"
      mask help:
      | A User-specified model may be selected as Controller or Dynamics of the vehicle. PreScan will copy the contents of the User-specified model into the user-specified model block.
      |
      | If update checkbox is checked the current user-specified model block will be deleted and will be REPLACED by (new) user specified model blocks. So, the current user specified model elements will be lost.
      |
      | Warning: If a new user-specified model is selected in the GUI, the user-specified model will be replaced.
      settings: DeleteFcn=PreScanBlockDeleteFcn;
      mask Help: eval('openHelp(227)')
      mask Display: userSpecifiedDynamics_mask_display();
  SELF_Demux : Subsystem  Tag=demux/SelfPort  mask(PreScan Demux Block:){}
      mask help:
      | The SELF port shows (state) information of the actor itself. The outputs are position in the experiment's axis system and the GPS coordinates, and the object's absolute velocity and compass heading.
      |
      | For more information, please click Help.
      settings: DeleteFcn=PreScanBlockDeleteFcn;
      mask Help: eval('openHelp(462)')
      mask Display:
      | port_label('output',1,'x [m]')
      | port_label('output',2,'y [m]')
      | port_label('output',3,'z [m]','texmode','on')
      | port_label('output',4,'Rotx [deg]','texmode','on')
      | port_label('output',5,'Roty [deg]','texmode','on')
      | port_label('output',6,'Rotz [deg]','texmode','on')
      | port_label('output',7,'GPS lat [deg]','texmode','on')
      | port_label('output',8,'GPS long [deg]','texmode','on')
      | port_label('output',9,'GPS alt [m]','texmode','on')
      | port_label('output',10,'Velocity [m/s]')
      | port_label('output',11,'Heading [deg]')
      | port_label('output',12,'Yaw rate [deg/s]')
  STATE_Audi_A8_Sedan_1_rc : RateTransition  Tag=mux_rc/StatePort  OutPortSampleTimeOpt=Inherit
  Terminator_{2..10} (9 alike) : Terminator
  To Workspace : ToWorkspace  VariableName=debug_control  SaveFormat=Timeseries  SampleTime=-1
  control module1 : Subsystem
  decision&planning module V0.1 : Subsystem  Commented=on
  decision&planning module with quad1 : Subsystem  Commented=on
  decision&planning module5.15 : Subsystem
  location module : Subsystem
  perception module : Subsystem
  routine module : Subsystem
  角度化为弧度 : Gain  Gain=pi/180
  角速度化为弧度制 : Gain  Gain=pi/180
  STATE_Audi_A8_Sedan_1_bus : Outport  Tag=outport/StatePort  OutDataTypeStr=Bus: PRESCAN_STATEACTUATORDATA  PortDimensions=1  SampleTime=50/1000
  wires:
  SELF_Demux/1(x [m]) -> [host_x]
  SELF_Demux/2(y [m]) -> [host_y]
  SELF_Demux/6(rotz [deg]) -> 角度化为弧度/1
  SELF_Demux/10(velocity [m/s]) -> [host_speed]
  SELF_Demux/12(yaw rate [deg/s]) -> 角速度化为弧度制/1
  角速度化为弧度制/1 -> [host_yaw_rate]
  角度化为弧度/1 -> [host_heading_xy]
  [lat_angle] -> Dynamics_UserSpecified/1(steer_sw)
  [throttle] -> Dynamics_UserSpecified/2(throttle)
  [brake] -> Dynamics_UserSpecified/3(brake)
  Dynamics_UserSpecified/3(vy) -> [host_vy]
  Dynamics_UserSpecified/4(ax) -> [host_ax]
  Dynamics_UserSpecified/5(ay) -> [host_ay]
  Dynamics_UserSpecified/2(vx) -> [host_vx]
  AIR_1_Demux/1(Range [m]) -> [sensor_range]
  AIR_1_Demux/2(Azimuth [deg]) -> [sensor_theta]
  AIR_1_Demux/5(Velocity [m/s]) -> [sensor_velocity]
  AIR_1_Demux/6(Heading [deg]) -> [sensor_heading]
  control module1/1(lateral_steer_sw) -> [lat_angle]
  [host_ay] -> location module/9(host_ay[m/s2])  "host_ay"
  location module/1(location info) -> perception module/1(location info), decision&planning module5.15/1(location info), control module1/1(location_info), [Location_info]
  [do_planning] -> decision&planning module5.15/Trigger
  [host_ax] -> location module/8(host_ax[m/s2])  "host_ax"
  [sensor_range] -> perception module/2(obs range)
  [planning_info] -> Delay/1
  control module1/2(throttle) -> [throttle]
  [host_speed] -> location module/7(host_speed[m/s])  "host_speed"
  [host_vy] -> location module/5(host_vy[m/s])  "host_vy"
  [time] -> control module1/4(current_time)
  Chart/1(do_planning()) -> [do_planning]
  [host_yaw_rate] -> location module/6(host_yawrate[rad/s])  "host_yawrate"
  [sensor_velocity] -> perception module/4(obs velocity)
  perception module/1(perception info) -> decision&planning module5.15/3(perception info)
  Constant3/1 -> control module1/3(control_predict_time[s])
  Clock/1 -> [time]
  routine module/1(global_path_info) -> decision&planning module5.15/2(routine info)
  [debug_control] -> To Workspace/1
  Delay/1 -> decision&planning module5.15/4(pre planning info)
  [sensor_heading] -> perception module/5(obs heading)
  Chart/2(do_control()) -> [do_control]
  [do_control] -> control module1/Trigger
  [sensor_theta] -> perception module/3(obs theta)
  [host_vx] -> location module/4(host_vx[m/s])  "host_vx"
  control module1/4(debug_control) -> [debug_control]
  [host_y] -> location module/2(host_y[m])  "host_y"
  decision&planning module5.15/1(planning_result) -> [planning_info], control module1/2(planning_result)
  control module1/3(brake) -> [brake]
  [host_x] -> location module/1(host_x[m])  "host_x"
  [time] -> decision&planning module5.15/5(current time)
  [host_heading_xy] -> location module/3(host_heading_xy[rad])  "host_heading_xy"
  STATE_Audi_A8_Sedan_1_rc/1 -> STATE_Audi_A8_Sedan_1_bus/1
  SELF_Audi_A8_Sedan_1/1 -> SELF_Demux/1(SELF)
  AIR_1/1 -> AIR_1_Demux/1(AIR)
  Dynamics_UserSpecified/1(State) -> STATE_Audi_A8_Sedan_1_rc/1
  AIR_1_Demux/3(Elevation [deg]) -> Terminator_10/1
  AIR_1_Demux/4(ID [-]) -> Terminator_2/1
  SELF_Demux/3(z [m]) -> Terminator_3/1
  SELF_Demux/4(rotx [deg]) -> Terminator_4/1
  SELF_Demux/5(roty [deg]) -> Terminator_5/1
  SELF_Demux/7(GPS lat [deg]) -> Terminator_6/1
  SELF_Demux/8(GPS long [deg]) -> Terminator_7/1
  SELF_Demux/9(GPS alt [m]) -> Terminator_8/1
  SELF_Demux/11(heading [deg]) -> Terminator_9/1

== system testEMplanner_cs/Box_1 ==
  SELF_Box_1 : Inport  Tag=inport/SelfPort  OutDataTypeStr=Bus: PRESCAN_SELFSENSORDATA  PortDimensions=1  SampleTime=50/1000  BusOutputAsStruct=on
  Dynamics_Empty : Subsystem  Tag=Dynamics_Empty
      mask Help: eval('openHelp(202)')
      mask Display: port_label('output', 1, 'State');text(0,0,' Empty\n')
  SELF_Demux : Subsystem  Tag=demux/SelfPort  mask(PreScan Demux Block:){}
      mask help:
      | The SELF port shows (state) information of the actor itself. The outputs are position in the experiment's axis system and the GPS coordinates, and the object's absolute velocity and compass heading.
      |
      | For more information, please click Help.
      settings: DeleteFcn=PreScanBlockDeleteFcn;
      mask Help: eval('openHelp(462)')
      mask Display:
      | port_label('output',1,'x [m]')
      | port_label('output',2,'y [m]')
      | port_label('output',3,'z [m]','texmode','on')
      | port_label('output',4,'Rotx [deg]','texmode','on')
      | port_label('output',5,'Roty [deg]','texmode','on')
      | port_label('output',6,'Rotz [deg]','texmode','on')
      | port_label('output',7,'GPS lat [deg]','texmode','on')
      | port_label('output',8,'GPS long [deg]','texmode','on')
      | port_label('output',9,'GPS alt [m]','texmode','on')
      | port_label('output',10,'Velocity [m/s]')
      | port_label('output',11,'Heading [deg]')
      | port_label('output',12,'Yaw rate [deg/s]')
  STATE_Box_1_rc : RateTransition  Tag=mux_rc/StatePort  OutPortSampleTimeOpt=Inherit
  Terminator_{1..12} (12 alike) : Terminator
  STATE_Box_1_bus : Outport  Tag=outport/StatePort  OutDataTypeStr=Bus: PRESCAN_STATEACTUATORDATA  PortDimensions=1  SampleTime=50/1000
  wires:
  STATE_Box_1_rc/1 -> STATE_Box_1_bus/1
  SELF_Box_1/1 -> SELF_Demux/1(SELF)
  Dynamics_Empty/1(State) -> STATE_Box_1_rc/1
  SELF_Demux/1(x [m]) -> Terminator_1/1
  SELF_Demux/2(y [m]) -> Terminator_2/1
  SELF_Demux/3(z [m]) -> Terminator_3/1
  SELF_Demux/4(rotx [deg]) -> Terminator_4/1
  SELF_Demux/5(roty [deg]) -> Terminator_5/1
  SELF_Demux/6(rotz [deg]) -> Terminator_6/1
  SELF_Demux/7(GPS lat [deg]) -> Terminator_7/1
  SELF_Demux/8(GPS long [deg]) -> Terminator_8/1
  SELF_Demux/9(GPS alt [m]) -> Terminator_9/1
  SELF_Demux/10(velocity [m/s]) -> Terminator_10/1
  SELF_Demux/11(heading [deg]) -> Terminator_11/1
  SELF_Demux/12(yaw rate [deg/s]) -> Terminator_12/1
